simulink model "chapter7_4"  (R2020a)
settings: Solver=VariableStepAuto  StartTime=0.0  StopTime=10.0  RelTol=1e-3
settings Model: Creator=ZUNAED  LastModifiedBy=ZUNAED

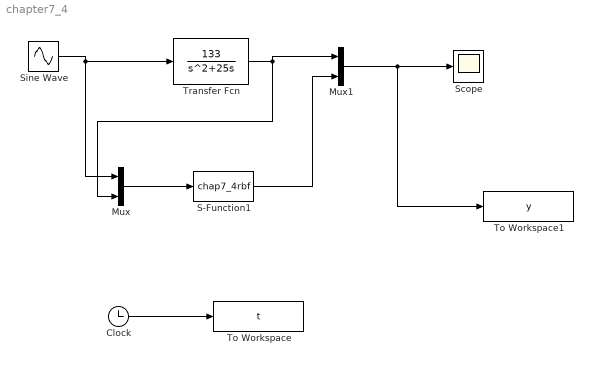
== system chapter7_4 ==
  Clock : Clock
  Mux : Mux  Inputs=2
  Mux1 : Mux  Inputs=2
  S-Function1 : S-Function  FunctionName=chap7_4rbf  SFunctionDeploymentMode=off  EnableBusSupport=off
  Scope : Scope
  Sine Wave : Sin  SampleTime=0.001
  To Workspace : ToWorkspace  VariableName=t  SaveFormat=Timeseries  SampleTime=-1
  To Workspace1 : ToWorkspace  VariableName=y  SaveFormat=Timeseries  SampleTime=-1
  Transfer Fcn : TransferFcn  Numerator=[133]  Denominator=[1 25 0]
  wires:
  Sine Wave/1 -> Transfer Fcn/1, Mux/1
  Clock/1 -> To Workspace/1
  Mux/1 -> S-Function1/1
  S-Function1/1 -> Mux1/2
  Mux1/1 -> To Workspace1/1, Scope/1
  Transfer Fcn/1 -> Mux1/1, Mux/2
